simulink model "sistema_control_observador"  (R2015b)
settings: Solver=VariableStepAuto  StartTime=0.0  StopTime=Tt  RelTol=1e-3
undefined symbols (not defined in the file): a, A11, A12, A21, A22, Ad, b, B1, B2, Bd, c, Cd, Dd, K, Kd, L, r, Ts, x1, x2, x3, x4
libraries: simulink x1
settings Model: Creator=pdoren  LastModifiedBy=pdoren
settings SolverCC: ZeroCrossAlgorithm=Adaptive

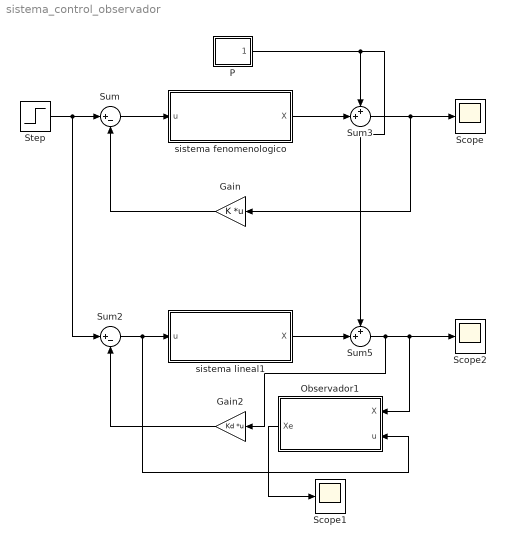
== system sistema_control_observador ==
  Gain : Gain  Gain=K  Multiplication=Matrix(K*u)
  Gain2 : Gain  Gain=Kd  Multiplication=Matrix(K*u)
  Observador1 : Subsystem
  P : Subsystem
  Scope : Scope
  Scope1 : Scope
  Scope2 : Scope
  Step : Step  After=r  SampleTime=0
  Sum : Sum  Inputs=|+-
  Sum2 : Sum  Inputs=|+-
  Sum3 : Sum  Inputs=++|
  Sum5 : Sum  Inputs=++|
  sistema fenomenologico : Subsystem
  sistema lineal1 : Subsystem
  wires:
  Sum/1 -> sistema fenomenologico/1(u)
  Step/1 -> Sum2/1, Sum/1
  Gain/1 -> Sum/2
  Sum2/1 -> Observador1/2(u), sistema lineal1/1(u)
  Gain2/1 -> Sum2/2
  sistema fenomenologico/1(X) -> Sum3/2
  sistema lineal1/1(X) -> Sum5/2
  Sum5/1 -> Gain2/1, Observador1/1(X), Scope2/1
  P/1(Out1) -> Sum3/1, Sum5/1
  Sum3/1 -> Gain/1, Scope/1
  Observador1/1(Xe) -> Scope1/1

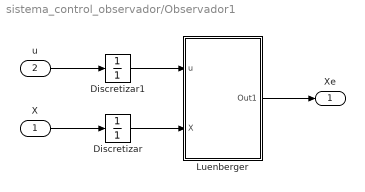
== system sistema_control_observador/Observador1 ==
  X : Inport
  u : Inport  Port=2
  Discretizar : DiscreteTransferFcn  Denominator=[1]  SampleTime=Ts
  Discretizar1 : DiscreteTransferFcn  Denominator=[1]  SampleTime=Ts
  Luenberger : Subsystem
  Xe : Outport
  wires:
  X/1 -> Discretizar/1
  Discretizar/1 -> Luenberger/2(X)
  u/1 -> Discretizar1/1
  Discretizar1/1 -> Luenberger/1(u)
  Luenberger/1(Out1) -> Xe/1

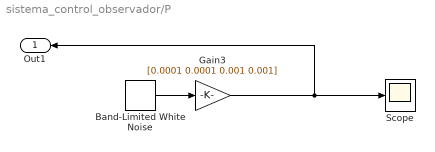
== system sistema_control_observador/P ==
  Band-Limited White Noise : simulink/Sources/Band-Limited White Noise  Cov=[0.01]  Ts=0.002  seed=[23341]
  Gain3 : Gain  Gain=[0.0001 0.0001 0.001 0.001]
  Scope : Scope
  Out1 : Outport
  wires:
  Gain3/1 -> Out1/1, Scope/1
  Band-Limited White Noise/1 -> Gain3/1

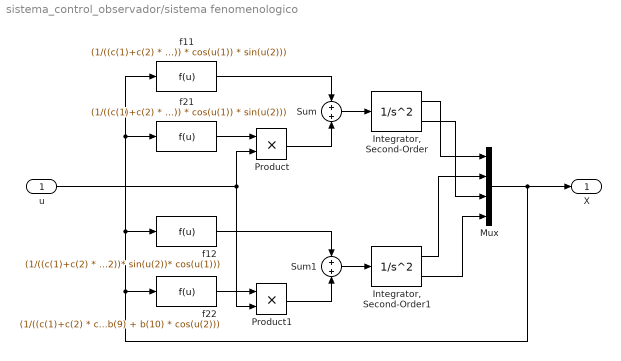
== system sistema_control_observador/sistema fenomenologico ==
  u : Inport
  "Integrator, Second-Order" : SecondOrderIntegrator  ICX=x1  ICDXDT=x3
  "Integrator, Second-Order1" : SecondOrderIntegrator  ICX=x2  ICDXDT=x4
  Mux : Mux
  Product : Product
  Product1 : Product
  Sum : Sum  Inputs=+|+
  Sum1 : Sum  Inputs=+|+
  f11 : Fcn  Expr=(1/((c(1)+c(2) * cos(u(2))^2) * c(3))) * ((a(1) + a(2) * cos(u(2))) * sin(u(2)) * u(3)^2 + a(3) * sin(u(2)) * u(4) * u(3) + a(4) * sin(u(2)) * u(4)^2 + (a(5) + a(6) * cos(u(2))) * u(4) + a(9) * sin(u(1)) * cos(u(2))^2 + a(10) * sin(u(1)) + a(11) * cos(u(2)) * cos(u(1)) * sin(u(2)))
  f12 : Fcn  Expr=(1/((c(1)+c(2) * cos(u(2))^2) * c(3))) * ((b(1) + b(2) * cos(u(2))) * sin(u(2)) * u(3)^2 + (b(3) * cos(u(2)) + b(4))* sin(u(2)) * u(4) * u(1) + (b(5) + b(6) * cos(u(2)))* sin(u(2)) * u(4)^2 + (b(7) + b(8)* cos(u(2))) * u(4) + (b(11) + b(12)* cos(u(2)))* sin(u(1)) + b(13) * sin(u(1)) * cos(u(2))^2 + b(14) * cos(u(1)) * sin(u(2)) + b(15) * cos(u(2))* sin(u(2))* cos(u(1)))
  f21 : Fcn  Expr=(1/((c(1)+c(2) * cos(u(2))^2) * c(3))) * ((a(1) + a(2) * cos(u(2))) * sin(u(2)) * u(3)^2 + a(3) * sin(u(2)) * u(4) * u(3) + a(4) * sin(u(2)) * u(4)^2 + (a(5) + a(6) * cos(u(2))) * u(4) + a(9) * sin(u(1)) * cos(u(2))^2 + a(10) * sin(u(1)) + a(11) * cos(u(2)) * cos(u(1)) * sin(u(2)))
  f22 : Fcn  Expr=(1/((c(1)+c(2) * cos(u(2))^2) * c(3))) * (b(9) + b(10) * cos(u(2)))
  X : Outport
  wires:
  Product/1 -> Sum/2
  f11/1 -> Sum/1
  f21/1 -> Product/1
  "Integrator, Second-Order"/1 -> Mux/1
  "Integrator, Second-Order1"/2 -> Mux/4
  Sum1/1 -> "Integrator, Second-Order1"/1
  "Integrator, Second-Order"/2 -> Mux/3
  "Integrator, Second-Order1"/1 -> Mux/2
  u/1 -> Product1/2, Product/2
  Mux/1 -> X/1, f22/1, f12/1, f21/1, f11/1
  Sum/1 -> "Integrator, Second-Order"/1
  f12/1 -> Sum1/1
  f22/1 -> Product1/1
  Product1/1 -> Sum1/2

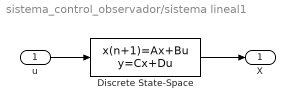
== system sistema_control_observador/sistema lineal1 ==
  u : Inport
  Discrete State-Space : DiscreteStateSpace  A=Ad  B=Bd  C=Cd  D=Dd  X0=[x1 x2 x3 x4]  SampleTime=Ts
  X : Outport
  wires:
  u/1 -> Discrete State-Space/1
  Discrete State-Space/1 -> X/1

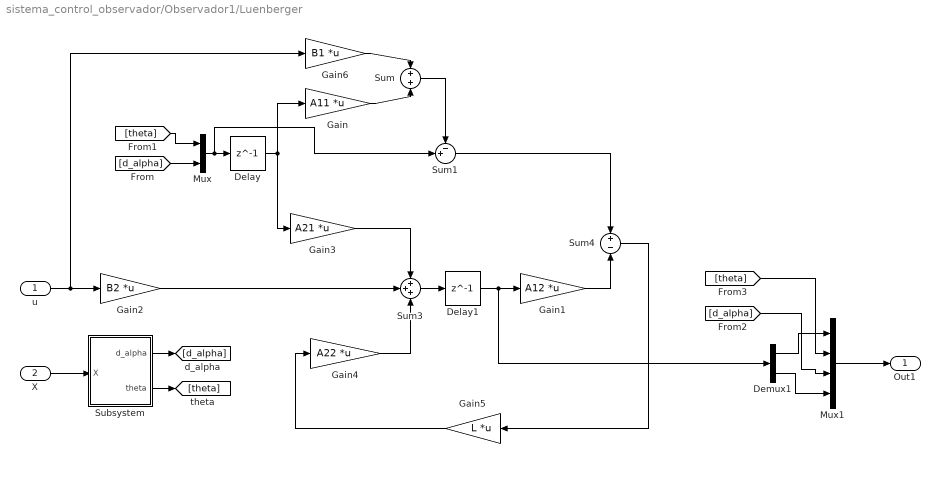
== system sistema_control_observador/Observador1/Luenberger ==
  u : Inport
  X : Inport  Port=2
  Delay : Delay  DelayLength=1
  Delay1 : Delay  DelayLength=1
  Demux1 : Demux  Outputs=2
  Gain : Gain  Gain=A11  Multiplication=Matrix(K*u)
  Gain1 : Gain  Gain=A12  Multiplication=Matrix(K*u)
  Gain2 : Gain  Gain=B2  Multiplication=Matrix(K*u)
  Gain3 : Gain  Gain=A21  Multiplication=Matrix(K*u)
  Gain4 : Gain  Gain=A22  Multiplication=Matrix(K*u)
  Gain5 : Gain  Gain=L  Multiplication=Matrix(K*u)
  Gain6 : Gain  Gain=B1  Multiplication=Matrix(K*u)
  Mux : Mux  Inputs=2
  Mux1 : Mux
  Subsystem : Subsystem
  Sum : Sum  Inputs=+|+
  Sum1 : Sum  Inputs=-+|
  Sum3 : Sum  Inputs=+++
  Sum4 : Sum  Inputs=+|-
  Out1 : Outport
  wires:
  Gain6/1 -> Sum/1
  Gain/1 -> Sum/2
  Sum4/1 -> Gain5/1
  u/1 -> Gain6/1, Gain2/1
  Gain2/1 -> Sum3/2
  Sum3/1 -> Delay1/1
  Mux1/1 -> Out1/1
  Sum/1 -> Sum1/1
  X/1 -> Subsystem/1(X)
  Gain3/1 -> Sum3/1
  Subsystem/2(theta) -> [theta]
  Subsystem/1(d_alpha) -> [d_alpha]
  [d_alpha] -> Mux/2
  [theta] -> Mux/1
  Gain1/1 -> Sum4/2
  Sum1/1 -> Sum4/1
  Delay1/1 -> Gain1/1, Demux1/1
  Mux/1 -> Sum1/2, Delay/1
  Delay/1 -> Gain3/1, Gain/1
  Gain4/1 -> Sum3/3
  Demux1/1 -> Mux1/1
  [d_alpha] -> Mux1/3
  Demux1/2 -> Mux1/4
  [theta] -> Mux1/2
  Gain5/1 -> Gain4/1

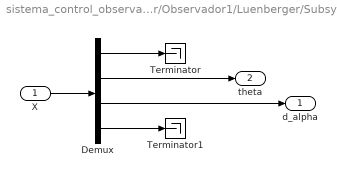
== system sistema_control_observador/Observador1/Luenberger/Subsystem ==
  X : Inport
  Demux : Demux
  Terminator : Terminator
  Terminator1 : Terminator
  d_alpha : Outport
  theta : Outport  Port=2
  wires:
  X/1 -> Demux/1
  Demux/2 -> theta/1
  Demux/3 -> d_alpha/1
  Demux/1 -> Terminator/1
  Demux/4 -> Terminator1/1
